simulink model "Resilient MPC"  (R2018b)
settings: Solver=VariableStepAuto  StartTime=0.0  StopTime=10  RelTol=1e-3
undefined symbols (not defined in the file or in its folder): a1, F, n1, Np, np, O, p, phi, sigbuilder_block, sigma, Ts
libraries: simulink x2
settings Model: Creator=lenovo  LastModifiedBy=lenovo
settings DebuggingCC: UnderSpecifiedDimensionMsg=warning

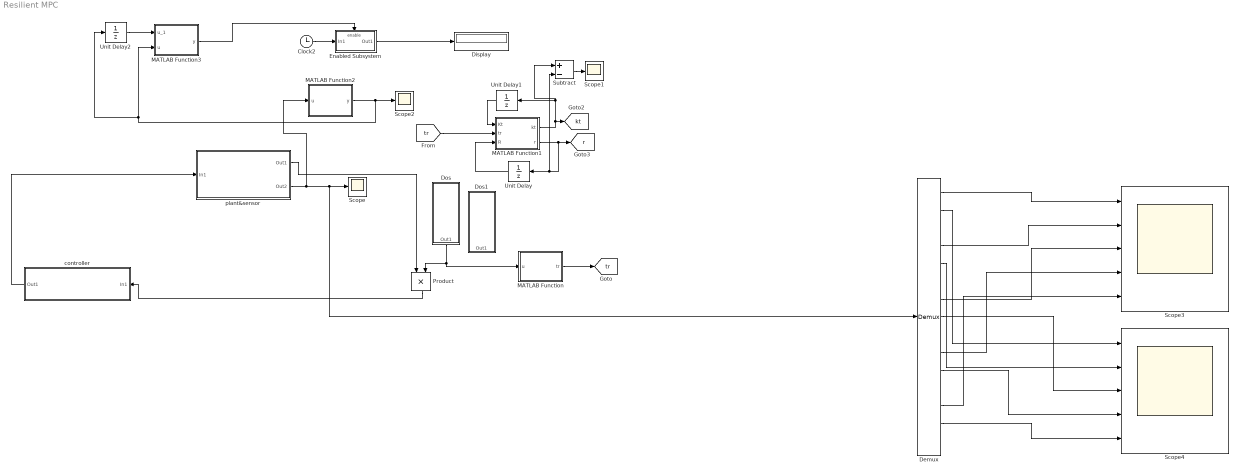
== system Resilient MPC ==
  Clock2 : Clock
  Demux : Demux  Outputs=15
  Display : Display
  Dos : Subsystem
  Dos1 : Subsystem
  Enabled Subsystem : Subsystem  TreatAsAtomicUnit=on
  MATLAB Function : MATLAB Function  TreatAsAtomicUnit=on
  MATLAB Function1 : MATLAB Function  TreatAsAtomicUnit=on
  MATLAB Function2 : MATLAB Function  TreatAsAtomicUnit=on
  MATLAB Function3 : MATLAB Function  TreatAsAtomicUnit=on
  Product : Product
  Scope : Scope
  Scope1 : Scope
  Scope2 : Scope
  Scope3 : Scope  NumInputPorts=5
  Scope4 : Scope  NumInputPorts=5
  Subtract : Sum  Inputs=+-
  Unit Delay : UnitDelay  SampleTime=0.1
  Unit Delay1 : UnitDelay  SampleTime=0.1
  Unit Delay2 : UnitDelay  SampleTime=0.1
  controller : Subsystem
  "plant&sensor " : Subsystem
  tag scope: kt=global, r=global, tr=global
  wires:
  MATLAB Function/1(tr) -> [tr]
  Unit Delay1/1 -> MATLAB Function1/1(Kt)
  "plant&sensor "/2(Out2) -> Demux/1, Scope/1, MATLAB Function2/1(u)
  MATLAB Function2/1(y) -> Unit Delay2/1, MATLAB Function3/2(u), Scope2/1
  Unit Delay/1 -> MATLAB Function1/3(R)
  MATLAB Function1/1(kt) -> Unit Delay1/1, Subtract/1, [kt]
  controller/1(Out1) -> "plant&sensor "/1(In1)
  Enabled Subsystem/1(Out1) -> Display/1
  Product/1 -> controller/1(In1)
  [tr] -> MATLAB Function1/2(tr)
  Subtract/1 -> Scope1/1
  MATLAB Function3/1(y) -> Enabled Subsystem/Enable
  Dos/1(Out1) -> MATLAB Function/1(u), Product/2
  Clock2/1 -> Enabled Subsystem/1(In1)
  MATLAB Function1/2(r) -> Subtract/2, Unit Delay/1, [r]
  Unit Delay2/1 -> MATLAB Function3/1(u_1)
  Demux/10 -> Scope3/4
  "plant&sensor "/1(Out1) -> Product/1
  Demux/1 -> Scope3/1
  Demux/2 -> Scope4/1
  Demux/13 -> Scope3/5
  Demux/7 -> Scope3/3
  Demux/8 -> Scope4/3
  Demux/5 -> Scope4/2
  Demux/4 -> Scope3/2
  Demux/11 -> Scope4/4
  Demux/14 -> Scope4/5

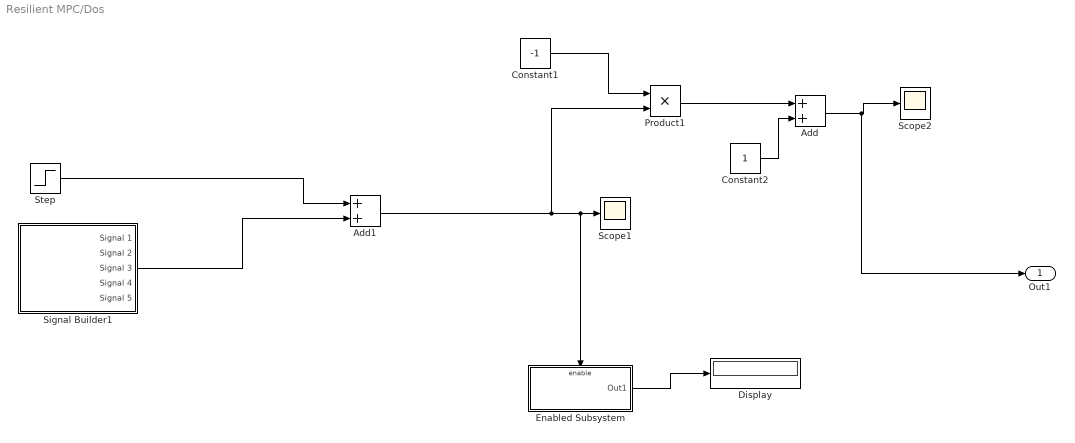
== system Resilient MPC/Dos ==
  Add : Sum
  Add1 : Sum
  Constant1 : Constant  Value=-1
  Constant2 : Constant
  Display : Display
  Enabled Subsystem : Subsystem  TreatAsAtomicUnit=on
  Product1 : Product
  Scope1 : Scope
  Scope2 : Scope
  Signal Builder1 : Subsystem  Tag=STV Subsys  LoadFcn=sigbuilder_block('load');  StartFcn=sigbuilder_block('start');  StopFcn=sigbuilder_block('stop');  ClipboardFcn=sigbuilder_block('clipboard');  mask(Sigbuilder block){tuvar=[0:10]}
      mask help: Simulink:masks:SigbuilderBlock_MD
      mask init:
      | if ~strcmp(get_param(bdroot(gcbh),'SimulationStatus'),'stopped') tuvar = sigbuilder_block('maskInit'); end
      settings: CopyFcn=sigbuilder_block('copy');  DeleteFcn=sigbuilder_block('delete');  ModelCloseFcn=sigbuilder_block('modelClose');  PreSaveFcn=sigbuilder_block('preSave');  PauseFcn=sigbuilder_block('pause');  ContinueFcn=sigbuilder_block('continue');  NameChangeFcn=sigbuilder_block('namechange');  OpenFcn=sigbuilder_block('open',[5.4 30 1141.2 522.6 ]);  CloseFcn=sigbuilder_block('close');
      mask Display: plot(0, 0, 100, 100,[2, 2, 32, 32, 2], [68, 8, 8, 68, 68],[32, 2], [38, 38], [32, 19, 2],[53, 60, 44], [32, 17, 17, 2],[16, 16, 31, 31]);txt = getActiveGroup(gcbh);text(2, 100, txt,'verticalAlignment', 'top');
  Step : Step  After=-1  SampleTime=10
  Out1 : Outport
  wires:
  Enabled Subsystem/1(Out1) -> Display/1
  Constant1/1 -> Product1/1
  Product1/1 -> Add/1
  Constant2/1 -> Add/2
  Add/1 -> Out1/1, Scope2/1
  Step/1 -> Add1/1
  Add1/1 -> Product1/2, Enabled Subsystem/Enable, Scope1/1
  Signal Builder1/3(Signal 3) -> Add1/2

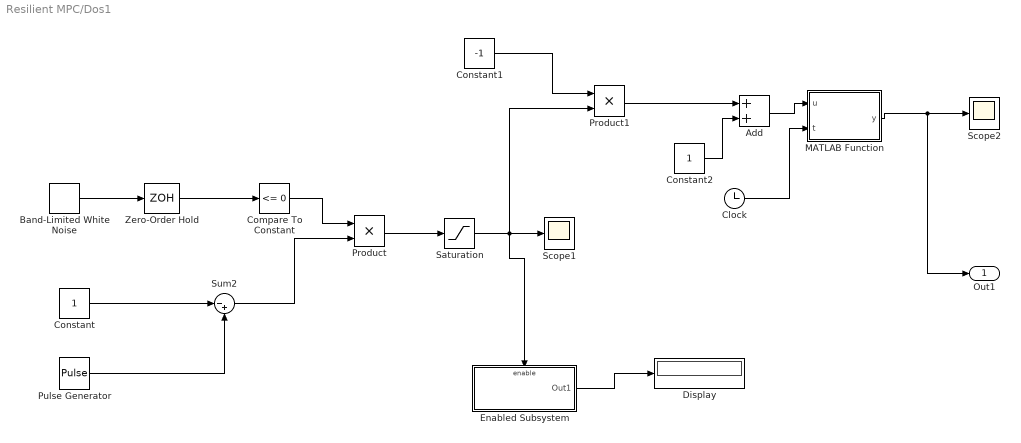
== system Resilient MPC/Dos1 ==
  Add : Sum
  Band-Limited White Noise : simulink/Sources/Band-Limited White Noise  Cov=[0.1]  Ts=0.1  seed=[23341]
  Clock : Clock
  Compare To Constant : simulink/Logic and Bit Operations/Compare To Constant  relop=<=  const=0  OutDataTypeStr=boolean
  Constant : Constant
  Constant1 : Constant  Value=-1
  Constant2 : Constant
  Display : Display
  Enabled Subsystem : Subsystem  TreatAsAtomicUnit=on
  MATLAB Function : MATLAB Function  TreatAsAtomicUnit=on
  Product : Product
  Product1 : Product
  Pulse Generator : DiscretePulseGenerator  PulseType=Time based  Amplitude=2  PulseWidth=50
  Saturation : Saturate  UpperLimit=1  LowerLimit=0
  Scope1 : Scope
  Scope2 : Scope
  Sum2 : Sum  Inputs=|-+
  Zero-Order Hold : ZeroOrderHold  SampleTime=-1
  Out1 : Outport
  wires:
  Compare To Constant/1 -> Product/1
  Saturation/1 -> Product1/2, Enabled Subsystem/Enable, Scope1/1
  Pulse Generator/1 -> Sum2/2
  Enabled Subsystem/1(Out1) -> Display/1
  Sum2/1 -> Product/2
  Band-Limited White Noise/1 -> Zero-Order Hold/1
  Zero-Order Hold/1 -> Compare To Constant/1
  Constant/1 -> Sum2/1
  Product/1 -> Saturation/1
  Constant1/1 -> Product1/1
  Product1/1 -> Add/1
  Constant2/1 -> Add/2
  Add/1 -> MATLAB Function/1(u)
  MATLAB Function/1(y) -> Out1/1, Scope2/1
  Clock/1 -> MATLAB Function/2(t)

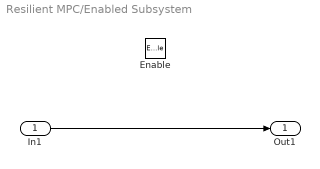
== system Resilient MPC/Enabled Subsystem ==
  In1 : Inport
  Enable : EnablePort
  Out1 : Outport
  wires:
  In1/1 -> Out1/1

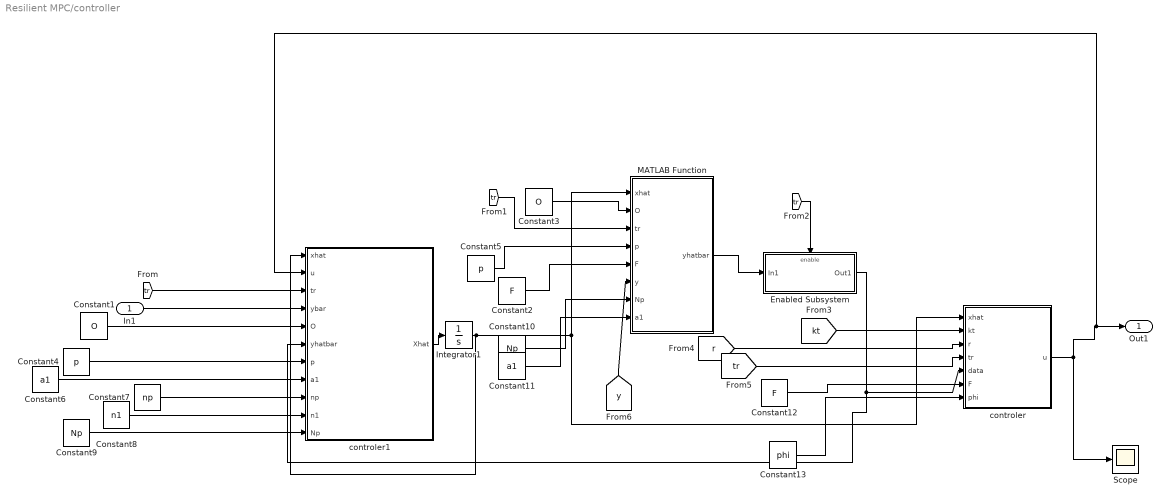
== system Resilient MPC/controller ==
  In1 : Inport
  Constant1 : Constant  Value=O
  Constant10 : Constant  Value=Np
  Constant11 : Constant  Value=a1
  Constant12 : Constant  Value=F
  Constant13 : Constant  Value=phi
  Constant2 : Constant  Value=F
  Constant3 : Constant  Value=O
  Constant4 : Constant  Value=p
  Constant5 : Constant  Value=p
  Constant6 : Constant  Value=a1
  Constant7 : Constant  Value=np
  Constant8 : Constant  Value=n1
  Constant9 : Constant  Value=Np
  Enabled Subsystem : Subsystem  TreatAsAtomicUnit=on
  Integrator1 : Integrator  InitialCondition=-10*[-7;-6;-5;-4;-3;-2;-1;0;1;2;3;4;5;6;7]
  MATLAB Function : MATLAB Function  TreatAsAtomicUnit=on
  Scope : Scope
  controler : MATLAB Function  TreatAsAtomicUnit=on
  controler1 : MATLAB Function  TreatAsAtomicUnit=on
  Out1 : Outport
  wires:
  controler1/1(Xhat) -> Integrator1/1
  controler/1(u) -> controler1/2(u), Out1/1, Scope/1
  [tr] -> controler1/3(tr)
  In1/1 -> controler1/4(ybar)
  Constant1/1 -> controler1/5(O)
  Constant3/1 -> MATLAB Function/2(O)
  [tr] -> MATLAB Function/3(tr)
  MATLAB Function/1(yhatbar) -> Enabled Subsystem/1(In1)
  [tr] -> Enabled Subsystem/Enable
  Enabled Subsystem/1(Out1) -> controler/5(data), controler1/6(yhatbar)
  [tr] -> controler/4(tr)
  [r] -> controler/3(r)
  [kt] -> controler/2(kt)
  Integrator1/1 -> controler1/1(xhat), MATLAB Function/1(xhat), controler/1(xhat)
  Constant2/1 -> MATLAB Function/5(F)
  Constant4/1 -> controler1/7(p)
  Constant5/1 -> MATLAB Function/4(p)
  [y] -> MATLAB Function/6(y)
  Constant6/1 -> controler1/8(a1)
  Constant7/1 -> controler1/9(np)
  Constant8/1 -> controler1/10(n1)
  Constant9/1 -> controler1/11(Np)
  Constant10/1 -> MATLAB Function/7(Np)
  Constant11/1 -> MATLAB Function/8(a1)
  Constant12/1 -> controler/6(F)
  Constant13/1 -> controler/7(phi)

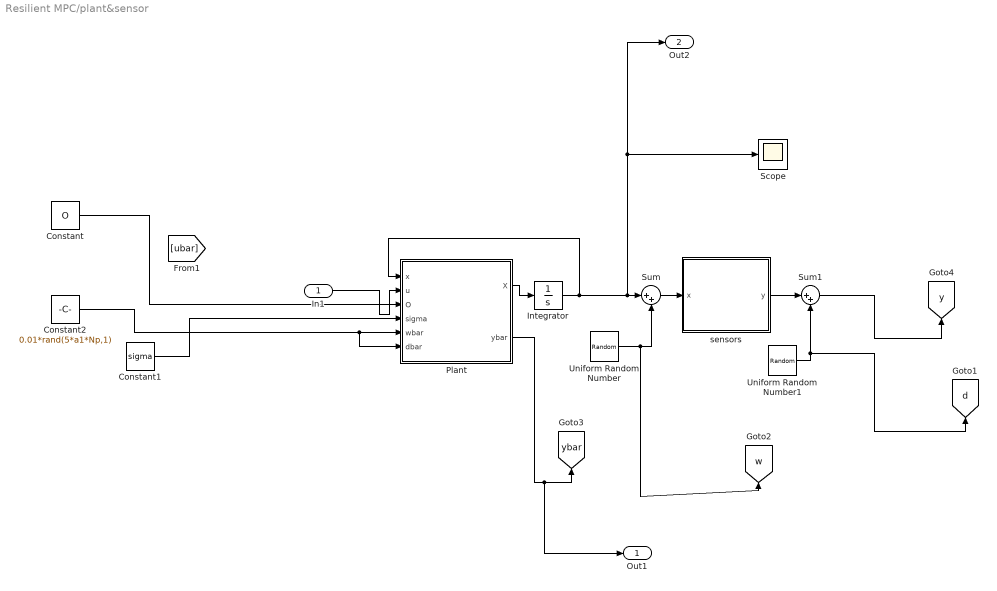
== system Resilient MPC/plant&sensor  ==
  In1 : Inport
  Constant : Constant  Value=O
  Constant1 : Constant  Value=sigma
  Constant2 : Constant  Value=0.01*rand(5*a1*Np,1)
  Integrator : Integrator  InitialCondition=10*[-7;-6;-5;-4;-3;-2;-1;0;1;2;3;4;5;6;7]
  Plant : MATLAB Function  TreatAsAtomicUnit=on
  Scope : Scope
  Sum : Sum  Inputs=|++
  Sum1 : Sum  Inputs=|++
  Uniform Random Number : UniformRandomNumber  Minimum=-0.01  Maximum=0.01  SampleTime=Ts
  Uniform Random Number1 : UniformRandomNumber  Minimum=-0.01  Maximum=0.01  SampleTime=Ts
  sensors : MATLAB Function  TreatAsAtomicUnit=on
  Out1 : Outport
  Out2 : Outport  Port=2
  tag scope: d=global, w=global, y=global, ybar=global
  wires:
  Sum/1 -> sensors/1(x)
  sensors/1(y) -> Sum1/1
  Uniform Random Number1/1 -> [d], Sum1/2
  Plant/1(X) -> Integrator/1
  Integrator/1 -> Out2/1, Scope/1, Sum/1, Plant/1(x)
  Uniform Random Number/1 -> [w], Sum/2
  In1/1 -> Plant/2(u)
  Constant/1 -> Plant/3(O)
  Constant1/1 -> Plant/4(sigma)
  Plant/2(ybar) -> Out1/1, [ybar]
  Constant2/1 -> Plant/6(dbar), Plant/5(wbar)
  Sum1/1 -> [y]

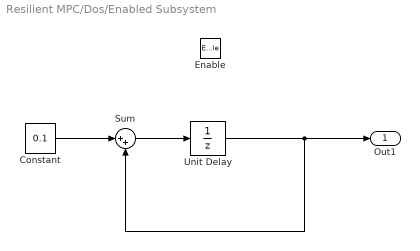
== system Resilient MPC/Dos/Enabled Subsystem ==
  Enable : EnablePort
  Constant : Constant  Value=0.1
  Sum : Sum  Inputs=|++
  Unit Delay : UnitDelay  SampleTime=-1
  Out1 : Outport
  wires:
  Unit Delay/1 -> Out1/1, Sum/2
  Constant/1 -> Sum/1
  Sum/1 -> Unit Delay/1

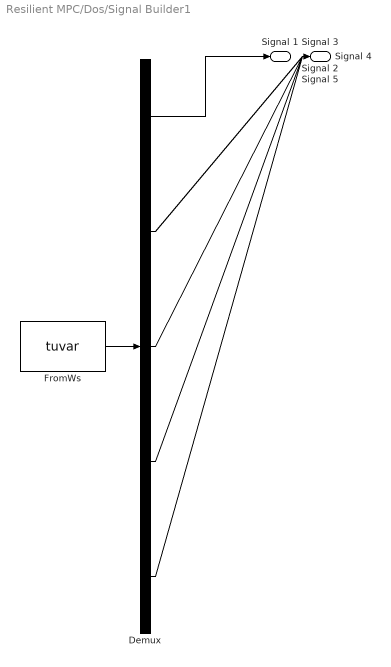
== system Resilient MPC/Dos/Signal Builder1 ==
  Demux : Demux  Tag=STV Demux  Outputs=5
  FromWs : FromWorkspace  Tag=STV FromWs  VariableName=tuvar  SampleTime=0
      SigBuilderData=|
      | common.afterFinalStr = 'Extrapolate'
      | common.sampleTime = 0
      | dataSet.timeRange = [0 10]
      | dataSet.name = 'Group 1'
      | sbobj.Groups.Name = 'Group 1'
      | sbobj.Groups.Signals(1).Name = 'Signal 1'
      | sbobj.Groups.Signals(1).XData = [0 4 4 6 6 10]
      | sbobj.Groups.Signals(1).YData = [0 0 1 1 0 0]
      | sbobj.Groups.Signals(2).Name = 'Signal 2'
      | sbobj.Groups.Signals(2).XData = [0 0.125 0.125 0.25 0.25 0.375 0.375 0.5 0.5 0.625 0.625 0.75 0.75 0.875 0.875 1 1 1.125 1.125 1.25 1.25 1.375 1.375 1.5 1.5 1.625 1.625 1.75 1.75 1.875 1.875 2 2 2.125 2.125 2.25 2.25 2.375 2.375 2.5 2.5 2.625 2.625 2.75 2.75 2.875 2.875 3 3 3.125 3.125 3.25 3.25 3.375 3.375 3.5 3.5 3.625 3.625 3.75 3.75 3.875 3.875 4 4 4.125 4.125 4.25 4.25 4.375 4.375 4.5 4.5 4.625 4.625 4.75 4.75 4.875 4.875 5 5 5.125 5.125 5.25 5.25 5.375 5.375 5.5 5.5 5.625 5.625 5.75 5.75 5.875 5.875 6 6 6.125 6.125 6.25 6.25 6.375 6.375 6.5 6.5 6.625 6.625 6.75 6.75 6.875 6.875 7 7 7.125 7.125 7.25 7.25 7.375 7.375 7.5 7.5 7.625 7.625 7.75 7.75 7.875 7.875 8 8 8.125 8.125 8.25 8.25 8.375 8.375 8.5 8.5 8.625 8.625 8.75 8.75 8.875 8.875 9 9 9.125 9.125 9.25 9.25 9.375 9.375 9.5 9.5 9.625 9.625 9.75 9.75 9.875 9.875 10]
      | sbobj.Groups.Signals(2).YData = [1 1 -1 -1 1 1 -1 -1 1 1 -1 -1 1 1 -1 -1 1 1 -1 -1 1 1 -1 -1 1 1 -1 -1 1 1 -1 -1 1 1 -1 -1 1 1 -1 -1 1 1 -1 -1 1 1 -1 -1 1 1 -1 -1 1 1 -1 -1 1 1 -1 -1 1 1 -1 -1 1 1 -1 -1 1 1 -1 -1 1 1 -1 -1 1 1 -1 -1 1 1 -1 -1 1 1 -1 -1 1 1 -1 -1 1 1 -1 -1 1 1 -1 -1 1 1 -1 -1 1 1 -1 -1 1 1 -1 -1 1 1 -1 -1 1 1 -1 -1 1 1 -1 -1 1 1 -1 -1 1 1 -1 -1 1 1 -1 -1 1 1 -1 -1 1 1 -1 -1 1 1 -1 -1 1 1 -1 -1 1 1 -1 -1 1 1 -1 -1]
      | sbobj.Groups.Signals(3).Name = 'Signal 3'
      | sbobj.Groups.Signals(3).XData = [0 0.16 0.16 0.333333333333 0.4 0.4 0.46 0.46 0.833333333333 1 1.005 1.005 1.3 1.3 1.8 1.8 1.9 1.9 2.4 2.4 2.55 2.55 2.625 2.785 2.83333333333 3 3.2 3.2 3.4 3.4 3.5 3.66666666667 3.83333333333 4 4 4.17 4.17 4.33333333333 4.5 4.8 4.8 4.85 4.85 5 5.16666666667 5.33333333333 5.33333333333 5.5 5.5 5.66666666667 5.83333333333 5.83333333333 6 6 6.16666666667 6.33333333333 6.5 6.5 6.66666666667 6.66666666667 6.83333333333 7 7 7.16666666667 7.16666666667 7.33333333333 7.5 7.66666666667 7.83333333333 7.83333333333 8 8 8.16666666667 8.33333333333 8.5 8.5 8.66666666667 8.66666666667 8.83333333333 9 9.16666666667 9.33333333333 9.33333333333 9.5 9.5 9.66666666667 9.83333333333 10]
      | sbobj.Groups.Signals(3).YData = [0 0 1 1 1 0 0 1 1 1 1 0 0 1 1 0 0 1 1 0 0 1 1 1 1 1 1 0 0 1 1 1 1 1 0 0 1 1 1 1 0 0 1 1 1 1 0 0 1 1 1 0 0 1 1 1 1 0 0 1 1 1 0.005 0.005 1 1 1 1 1 0 0 1 1 1 1 0 0 1 1 1 1 1 0 0 1 1 1 1]
      | sbobj.Groups.Signals(4).Name = 'Signal 4'
      | sbobj.Groups.Signals(4).XData = [0 5 5 10]
      | sbobj.Groups.Signals(4).YData = [0 0 1 1]
      | sbobj.Groups.Signals(5).Name = 'Signal 5'
      | sbobj.Groups.Signals(5).XData = [0 0.45 0.45 0.5 0.5 0.95 0.95 1 1 1.45 1.45 1.5 1.5 1.95 1.95 2 2 2.45 2.45 2.5 2.5 2.95 2.95 3 3 3.45 3.45 3.5 3.5 3.95 3.95 4 4 4.45 4.45 4.5 4.5 4.95 4.95 5 5 5.45 5.45 5.5 5.5 5.95 5.95 6 6 6.45 6.45 6.5 6.5 6.95 6.95 7 7 7.45 7.45 7.5 7.5 7.95 7.95 8 8 8.45 8.45 8.5 8.5 8.95 8.95 9 9 9.45 9.45 9.5 9.5 9.95 9.95 10]
      | sbobj.Groups.Signals(5).YData = [1 1 0 0 1 1 0 0 1 1 0 0 1 1 0 0 1 1 0 0 1 1 0 0 1 1 0 0 1 1 0 0 1 1 0 0 1 1 0 0 1 1 0 0 1 1 0 0 1 1 0 0 1 1 0 0 1 1 0 0 1 1 0 0 1 1 0 0 1 1 0 0 1 1 0 0 0.995 0.995 0 0]
  Signal 1 : Outport  Tag=STV Outport
  Signal 2 : Outport  Tag=STV Outport  Port=2
  Signal 3 : Outport  Tag=STV Outport  Port=3
  Signal 4 : Outport  Tag=STV Outport  Port=4
  Signal 5 : Outport  Tag=STV Outport  Port=5
  wires:
  Demux/1 -> Signal 1/1
  FromWs/1 -> Demux/1
  Demux/2 -> Signal 2/1
  Demux/3 -> Signal 3/1
  Demux/4 -> Signal 4/1
  Demux/5 -> Signal 5/1

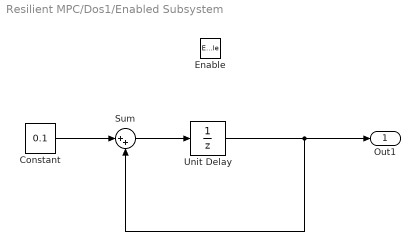
== system Resilient MPC/Dos1/Enabled Subsystem ==
  Enable : EnablePort
  Constant : Constant  Value=0.1
  Sum : Sum  Inputs=|++
  Unit Delay : UnitDelay  SampleTime=-1
  Out1 : Outport
  wires:
  Unit Delay/1 -> Out1/1, Sum/2
  Constant/1 -> Sum/1
  Sum/1 -> Unit Delay/1

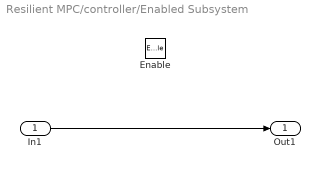
== system Resilient MPC/controller/Enabled Subsystem ==
  In1 : Inport
  Enable : EnablePort
  Out1 : Outport
  wires:
  In1/1 -> Out1/1

== matlab function Resilient MPC/controller/controler ==
  data: xhat input; u output; kt input; r input; tr input; data input; F input; phi input
function u = fcn(xhat,kt,r,tr, data,F,phi)
A=[ 1.049     0.03183    -0.02926
     0.01347       1.023  -0.0001932
  -0.0007729     -0.1155      0.9048];
B=[0.2026  6.946e-05
   -0.1504     0.1012
  0.008724    0.08931 ];
C=eye(3);

%  K=[    1.9115   -1.1429    0.4148
%     3.0186    4.4625   -0.5557];
q1=[1.9115   -1.1429    0.4148    0.0000    0.0000   -0.0000    0.0000    0.0000   -0.0000
    3.0186    4.4625   -0.5557   -0.0000   -0.0000    0.0000   -0.0000   -0.0000    0.0000
    0.0000    0.0000   -0.0000    1.9115   -1.1429    0.4148    0.0000    0.0000   -0.0000
   -0.0000   -0.0000    0.0000    3.0186    4.4625   -0.5557   -0.0000   -0.0000    0.0000
    0.0000    0.0000   -0.0000    0.0000    0.0000   -0.0000    1.9115   -1.1429    0.4148
   -0.0000   -0.0000    0.0000   -0.0000   -0.0000    0.0000    3.0186    4.4625   -0.5557
    0.0000    0.0000   -0.0000    0.0000    0.0000    0.0000    0.0000    0.0000   -0.0000
    0.0000    0.0000   -0.0000    0.0000    0.0000   -0.0000   -0.0000   -0.0000    0.0000
    0.0000    0.0000   -0.0000   -0.0000   -0.0000    0.0000   -0.0000   -0.0000    0.0000
    0.0000    0.0000   -0.0000    0.0000    0.0000   -0.0000    0.0000    0.0000   -0.0000
];
q2=[-0.0000   -0.0000    0.0000   -0.0000   -0.0000    0.0000
    0.0000    0.0000   -0.0000    0.0000    0.0000    0.0000
    0.0000    0.0000   -0.0000   -0.0000   -0.0000    0.0000
   -0.0000   -0.0000    0.0000    0.0000    0.0000   -0.0000
    0.0000    0.0000   -0.0000    0.0000    0.0000   -0.0000
   -0.0000   -0.0000    0.0000    0.0000    0.0000   -0.0000
    1.9115   -1.1429    0.4148   -0.0000   -0.0000    0.0000
    3.0186    4.4625   -0.5557   -0.0000   -0.0000    0.0000
    0.0000    0.0000   -0.0000    1.9115   -1.1429    0.4148
   -0.0000   -0.0000    0.0000    3.0186    4.4625   -0.5557
];

% if tr==1
%      K=[    1.9115   -1.1429    0.4148
%   3.0186    4.4625   -0.5557];
% K1=[eye(2) zeros(2,10)]*pinv(F'*F+0.1*eye(12))*(F'*phi);
% ee=data-C*xhat;
% e=[ee;zeros(15,1)];
K=[q1 q2];
  u=-K*xhat;
% else
%      K=[ 1.3140   -0.4724    0.1424
%     1.0121    1.3585    0.6980];
% u=-K*xhat;
%  end

== matlab function Resilient MPC/controller/controler1 ==
  data: xhat input; u input; Xhat output; tr input; ybar input; O input; yhatbar input; p input; a1 input; np input; n1 input; Np input
function Xhat = fcn(xhat,u,tr,ybar,O,yhatbar,p,a1,np,n1,Np)

A=[.48 .29 -.3;.13 .23 0;0 -1.2 -1];
B=[2 0;-1.5 1; 0 1];
C=eye(3);


A_bar=[ 1.049     0.03183    -0.02926
    0.01347       1.023  -0.0001932
    -0.0007729     -0.1155      0.9048];
B_bar=[0.2026  6.946e-05
    -0.1504     0.1012
    0.008724    0.08931 ];


G=[ 5.0468    1.5160   -0.5215
    1.5160    1.8633   -0.6870
    -0.5215   -0.6870    1.1919];
Gsigma=[G,zeros(a1,a1*Np-a1)];
Fbar=[B_bar zeros(a1,2*Np-2)];
A0=kron(eye(5),A);
B0=kron(eye(5),B);
C0=kron(eye(5),C);
G0=kron(eye(5),G);
Fbar0=kron(eye(5),Fbar);
Gsigma0=kron(eye(5),Gsigma);
O0=kron(eye(5),O);
if tr==1
    FF=p;
    ubar=FF*xhat;
    Xhat=A0*xhat+Fbar0*ubar+Gsigma0*(ybar-O0*xhat);
else
    Xhat=A0*xhat+B0*u+G0*(yhatbar-C0*xhat);
end

== matlab function Resilient MPC/controller/MATLAB Function ==
  data: xhat input; yhatbar output; O input; tr input; p input; F input; y input; Np input; a1 input
function yhatbar = fcn(xhat,O,tr,p,F,y,Np,a1)

FF=p;
ubar=FF*xhat;
F0=kron(eye(5),F);
O0=kron(eye(5),O);
if tr==1
yhatbar=y;
else
    H=[eye(3) zeros(3,Np*a1-a1)];
    H0=kron(eye(5),H);
yhatbar =H0*(O0*xhat+F0*ubar);
end

== matlab function Resilient MPC/MATLAB Function ==
  data: u input; tr output
function tr = fcn(u)
if u==1
    tr=1
else
    tr=0
end

== matlab function Resilient MPC/MATLAB Function3 ==
  data: u_1 input; u input; y output
function y = fcn(u_1,u)
if (u-u_1<.001)
y=0;
else
y=1;
end

== matlab function Resilient MPC/plant&sensor /Plant ==
  data: x input; u input; X output; O input; sigma input; wbar input; dbar input; ybar output
function [X,ybar] = fcn(x,u,O,sigma,wbar,dbar)
A=[.48 .29 -.3;.13 .23 0;0 -1.2 -1];
B=[2 0;-1.5 1; 0 1];
A0=kron(eye(5),A);
B0=kron(eye(5),B);
O0=kron(eye(5),O);
sigma0=kron(eye(5),sigma)
X =A0*x+B0*u;
ybar = O0*x+sigma0*wbar+dbar;

== matlab function Resilient MPC/plant&sensor /sensors ==
  data: x input; y output
function y = fcn(x)
C=eye(3);
C0=kron(eye(5),C);
y=C0*x;

== matlab function Resilient MPC/MATLAB Function2 ==
  data: u input; y output
function y = fcn( u)
y=norm(u);

== matlab function Resilient MPC/Dos1/MATLAB Function ==
  data: u input; y output; t input
function y = fcn(u,t)
if t>10
    y=1;
else
    y=u;
end

== matlab function Resilient MPC/MATLAB Function1 ==
  data: kt output; Kt input; tr input; r output; R input
function [kt,r] = fcn( Kt,tr,R)

kt=Kt+1;
if tr==1
    r=R+1;
else
    r=R;
end
